simulink model "MyoGesture6CH_UI"  (R2018b)
settings: Solver=VariableStepAuto  StartTime=0.0  StopTime=inf  RelTol=1e-3
undefined symbols (not defined in the file or in its folder): serial
libraries: dspstat3 x8, instrumentlib x2, aerolibanimutils x1, dspnetwork x1
settings Model: Creator=Bruger  LastModifiedBy=anton

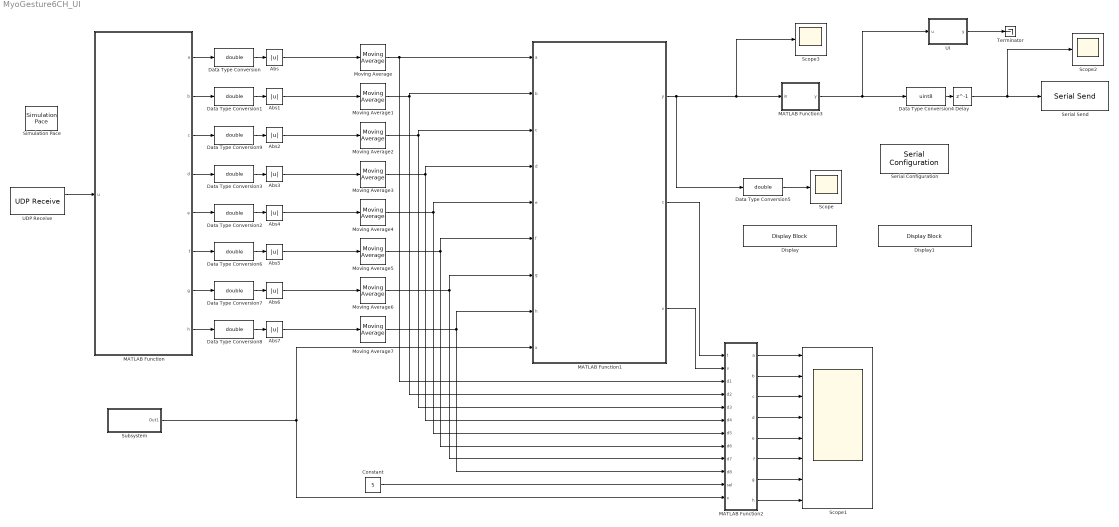
== system MyoGesture6CH_UI ==
  Abs{,1..7} (8 alike) : Abs
  Constant : Constant  Value=5
  Data Type Conversion{,1..3,5..9} (9 alike) : DataTypeConversion  OutDataTypeStr=double
  Data Type Conversion4 : DataTypeConversion  OutDataTypeStr=uint8
  Delay : Delay  DelayLength=1  InitialCondition=0
  Display : DisplayBlock  WebBlockId=99  LabelPosition=Hide
  Display1 : DisplayBlock  WebBlockId=154  LabelPosition=Hide
  MATLAB Function : MATLAB Function  TreatAsAtomicUnit=on
  MATLAB Function1 : MATLAB Function  TreatAsAtomicUnit=on
  MATLAB Function2 : MATLAB Function  TreatAsAtomicUnit=on
  MATLAB Function3 : MATLAB Function  TreatAsAtomicUnit=on
  Moving Average{,1..7} (8 alike) : dspstat3/Moving Average  Method=Sliding window  ForgettingFactorPort=off  SpecifyWindowLength=on  WindowLength=50  ForgettingFactor=0.9  SimulateUsing=Code generation
  Scope : Scope
  Scope1 : Scope  NumInputPorts=8
  Scope2 : Scope
  Scope3 : Scope
  Serial Configuration : instrumentlib/Serial Configuration  Priority=-200000  ComPortMenu=COM13  ComPort=COM13  ObjConstructor=serial('COM13');  BaudRate=12000000  DataBits=8  Parity=none  StopBits=1  FlowControl=none  Timeout=10  ByteOrder=LittleEndian
  Serial Send : instrumentlib/Serial Send  ComPortMenu=COM13  ComPort=COM13  ObjConstructor=serial('COM13');  Terminator=<none>  EnableBlockingMode=on
  Simulation Pace : aerolibanimutils/Simulation Pace  SimulationPace=1  SleepMode=Auto  OutputPaceError=off  SampleTime=1/30
  Subsystem : Subsystem
  Terminator : Terminator
  UDP Receive : dspnetwork/UDP Receive  localURL='0.0.0.0'  localPort=54000  remoteURL='0.0.0.0'  remotePort=-1  recvBufferSize=32  dims=255  signalDatatype=int8  isVarSize=off  showBlockingTime=off  blockingTime=0  sampletime=0.02  blockPlatform=[]
      settings: SourceProductName=DSP System Toolbox  SourceProductBaseCode=DS
  UI : MATLAB Function  Tag=rand  TreatAsAtomicUnit=on
  wires:
  UDP Receive/1 -> MATLAB Function/1(u)
  MATLAB Function/1(a) -> Data Type Conversion/1
  Data Type Conversion1/1 -> Abs1/1
  MATLAB Function/2(b) -> Data Type Conversion1/1
  Data Type Conversion2/1 -> Abs4/1
  Data Type Conversion3/1 -> Abs3/1
  Data Type Conversion6/1 -> Abs5/1
  Data Type Conversion7/1 -> Abs6/1
  Data Type Conversion8/1 -> Abs7/1
  Data Type Conversion9/1 -> Abs2/1
  MATLAB Function/8(h) -> Data Type Conversion8/1
  MATLAB Function/7(g) -> Data Type Conversion7/1
  MATLAB Function/6(f) -> Data Type Conversion6/1
  MATLAB Function/5(e) -> Data Type Conversion2/1
  MATLAB Function/4(d) -> Data Type Conversion3/1
  MATLAB Function/3(c) -> Data Type Conversion9/1
  Abs1/1 -> Moving Average1/1
  Abs7/1 -> Moving Average7/1
  Abs6/1 -> Moving Average6/1
  Abs5/1 -> Moving Average5/1
  Abs4/1 -> Moving Average4/1
  Abs3/1 -> Moving Average3/1
  Abs2/1 -> Moving Average2/1
  Moving Average1/1 -> MATLAB Function2/4(d2), MATLAB Function1/2(b)
  Moving Average2/1 -> MATLAB Function2/5(d3), MATLAB Function1/3(c)
  Moving Average3/1 -> MATLAB Function2/6(d4), MATLAB Function1/4(d)
  Moving Average4/1 -> MATLAB Function2/7(d5), MATLAB Function1/5(e)
  Moving Average5/1 -> MATLAB Function2/8(d6), MATLAB Function1/6(f)
  Moving Average6/1 -> MATLAB Function2/9(d7), MATLAB Function1/7(g)
  Moving Average7/1 -> MATLAB Function2/10(d8), MATLAB Function1/8(h)
  Data Type Conversion/1 -> Abs/1
  Abs/1 -> Moving Average/1
  Moving Average/1 -> MATLAB Function2/3(d1), MATLAB Function1/1(a)
  Subsystem/1(Out1) -> MATLAB Function1/9(x), MATLAB Function2/12(x)
  Constant/1 -> MATLAB Function2/11(sel)
  MATLAB Function2/8(h) -> Scope1/8
  MATLAB Function2/7(g) -> Scope1/7
  MATLAB Function2/1(a) -> Scope1/1
  MATLAB Function2/2(b) -> Scope1/2
  MATLAB Function2/3(c) -> Scope1/3
  MATLAB Function2/4(d) -> Scope1/4
  MATLAB Function2/5(e) -> Scope1/5
  MATLAB Function2/6(f) -> Scope1/6
  MATLAB Function1/2(t) -> MATLAB Function2/1(t)
  MATLAB Function1/3(v) -> MATLAB Function2/2(v)
  Data Type Conversion5/1 -> Scope/1
  Data Type Conversion4/1 -> Delay/1
  MATLAB Function1/1(y) -> Data Type Conversion5/1, Scope3/1, MATLAB Function3/1(in)
  Delay/1 -> Scope2/1, Serial Send/1
  MATLAB Function3/1(y) -> UI/1(u), Data Type Conversion4/1
  UI/1(y) -> Terminator/1

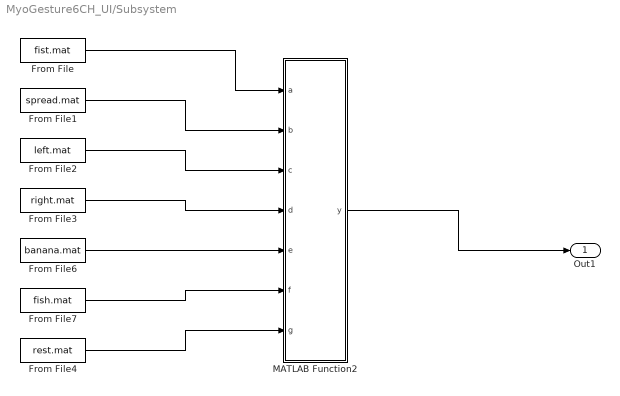
== system MyoGesture6CH_UI/Subsystem ==
  From File : FromFile  FileName=fist.mat  OutDataTypeStr=double  SampleTime=0  ExtrapolationBeforeFirstDataPoint=Hold first value  InterpolationWithinTimeRange=Zero order hold  ExtrapolationAfterLastDataPoint=Hold last value
  From File1 : FromFile  FileName=spread.mat  OutDataTypeStr=double  SampleTime=0  ExtrapolationBeforeFirstDataPoint=Hold first value  InterpolationWithinTimeRange=Zero order hold  ExtrapolationAfterLastDataPoint=Hold last value
  From File2 : FromFile  FileName=left.mat  OutDataTypeStr=double  SampleTime=0  ExtrapolationBeforeFirstDataPoint=Hold first value  InterpolationWithinTimeRange=Zero order hold  ExtrapolationAfterLastDataPoint=Hold last value
  From File3 : FromFile  FileName=right.mat  OutDataTypeStr=double  SampleTime=0  ExtrapolationBeforeFirstDataPoint=Hold first value  InterpolationWithinTimeRange=Zero order hold  ExtrapolationAfterLastDataPoint=Hold last value
  From File4 : FromFile  FileName=rest.mat  OutDataTypeStr=double  SampleTime=0  ExtrapolationBeforeFirstDataPoint=Hold first value  InterpolationWithinTimeRange=Zero order hold  ExtrapolationAfterLastDataPoint=Hold last value
  From File6 : FromFile  FileName=banana.mat  OutDataTypeStr=double  SampleTime=0  ExtrapolationBeforeFirstDataPoint=Hold first value  InterpolationWithinTimeRange=Zero order hold  ExtrapolationAfterLastDataPoint=Hold last value
  From File7 : FromFile  FileName=fish.mat  OutDataTypeStr=double  SampleTime=0  ExtrapolationBeforeFirstDataPoint=Hold first value  InterpolationWithinTimeRange=Zero order hold  ExtrapolationAfterLastDataPoint=Hold last value
  MATLAB Function2 : MATLAB Function  TreatAsAtomicUnit=on
  Out1 : Outport
  wires:
  MATLAB Function2/1(y) -> Out1/1
  From File/1 -> MATLAB Function2/1(a)
  From File6/1 -> MATLAB Function2/5(e)
  From File1/1 -> MATLAB Function2/2(b)
  From File7/1 -> MATLAB Function2/6(f)
  From File3/1 -> MATLAB Function2/4(d)
  From File2/1 -> MATLAB Function2/3(c)
  From File4/1 -> MATLAB Function2/7(g)

== matlab function MyoGesture6CH_UI/MATLAB Function1 ==
  data: a input; y output; b input; c input; d input; e input; f input; g input; h input; x input; t output; v output
function [y,t,v] = fcn(a,b,c,d,e,f,g,h,x)

%Percentage
t = 1.5; %top
v = 0.6; %bot

%constant
n = 1;  %top
m = 0;  %bot

    if a<x(1,7)*t+n & a>x(2,7)*v-m & b<x(3,7)*t+n & b>x(4,7)*v-m & c<x(5,7)*t+n & c>x(6,7)*v-m & d<x(7,7)*t+n & d>x(8,7)*v-m & e<x(9,7)*t+n & e>x(10,7)*v-m & f<x(11,7)*t+n & f>x(12,7)*v-m & g<x(13,7)*t+n & g>x(14,7)*v-m & h<x(15,7)*t+n & h>x(16,7)*v-m 
        y=0;
    elseif a<x(1,1)*t+n & a>x(2,1)*v-m & b<x(3,1)*t+n & b>x(4,1)*v-m & c<x(5,1)*t+n & c>x(6,1)*v-m & d<x(7,1)*t+n & d>x(8,1)*v-m & e<x(9,1)*t+n & e>x(10,1)*v-m & f<x(11,1)*t+n & f>x(12,1)*v-m & g<x(13,1)*t+n & g>x(14,1)*v-m & h<x(15,1)*t+n & h>x(16,1)*v-m 
        y=1;
    elseif a<x(1,2)*t+n & a>x(2,2)*v-m & b<x(3,2)*t+n & b>x(4,2)*v-m & c<x(5,2)*t+n & c>x(6,2)*v-m & d<x(7,2)*t+n & d>x(8,2)*v-m & e<x(9,2)*t+n & e>x(10,2)*v-m & f<x(11,2)*t+n & f>x(12,2)*v-m & g<x(13,2)*t+n & g>x(14,2)*v-m & h<x(15,2)*t+n & h>x(16,2)*v-m 
        y=2;
    elseif a<x(1,3)*t+n & a>x(2,3)*v-m & b<x(3,3)*t+n & b>x(4,3)*v-m & c<x(5,3)*t+n & c>x(6,3)*v-m & d<x(7,3)*t+n & d>x(8,3)*v-m & e<x(9,3)*t+n & e>x(10,3)*v-m & f<x(11,3)*t+n & f>x(12,3)*v-m & g<x(13,3)*t+n & g>x(14,3)*v-m & h<x(15,3)*t+n & h>x(16,3)*v-m 
        y=3;
    elseif a<x(1,4)*t+n & a>x(2,4)*v-m & b<x(3,4)*t+n & b>x(4,4)*v-m & c<x(5,4)*t+n & c>x(6,4)*v-m & d<x(7,4)*t+n & d>x(8,4)*v-m & e<x(9,4)*t+n & e>x(10,4)*v-m & f<x(11,4)*t+n & f>x(12,4)*v-m & g<x(13,4)*t+n & g>x(14,4)*v-m & h<x(15,4)*t+n & h>x(16,4)*v-m 
        y=4;
    elseif a<x(1,5)*t+n & a>x(2,5)*v-m & b<x(3,5)*t+n & b>x(4,5)*v-m & c<x(5,5)*t+n & c>x(6,5)*v-m & d<x(7,5)*t+n & d>x(8,5)*v-m & e<x(9,5)*t+n & e>x(10,5)*v-m & f<x(11,5)*t+n & f>x(12,5)*v-m & g<x(13,5)*t+n & g>x(14,5)*v-m & h<x(15,5)*t+n & h>x(16,5)*v-m 
        y=5;
%     elseif a<x(1,6)*t+n & a>x(2,6)*v-m & b<x(3,6)*t+n & b>x(4,6)*v-m & c<x(5,6)*t+n & c>x(6,6)*v-m & d<x(7,6)*t+n & d>x(8,6)*v-m & e<x(9,6)*t+n & e>x(10,6)*v-m & f<x(11,6)*t+n & f>x(12,6)*v-m & g<x(13,6)*t+n & g>x(14,6)*v-m & h<x(15,6)*t+n & h>x(16,6)*v-m 
%         y=6;
               
    else
y=0
    
    end

% %Threshold with Addition
% t = 9;
% v = 3;
% 
%     if a<x(1,1)+t & a>x(2,1)-v & b<x(3,1)+t & b>x(4,1)-v & c<x(5,1)+t & c>x(6,1)-v & d<x(7,1)+t & d>x(8,1)-v & e<x(9,1)+t & e>x(10,1)-v & f<x(11,1)+t & f>x(12,1)-v & g<x(13,1)+t & g>x(14,1)-v & h<x(15,1)+t & h>x(16,1)-v 
%         y=1;
%     elseif a<x(1,2)+t & a>x(2,2)-v & b<x(3,2)+t & b>x(4,2)-v & c<x(5,2)+t & c>x(6,2)-v & d<x(7,2)+t & d>x(8,2)-v & e<x(9,2)+t & e>x(10,2)-v & f<x(11,2)+t & f>x(12,2)-v & g<x(13,2)+t & g>x(14,2)-v & h<x(15,2)+t & h>x(16,2)-v 
%         y=2;
%     elseif a<x(1,3)+t & a>x(2,3)-v & b<x(3,3)+t & b>x(4,3)-v & c<x(5,3)+t & c>x(6,3)-v & d<x(7,3)+t & d>x(8,3)-v & e<x(9,3)+t & e>x(10,3)-v & f<x(11,3)+t & f>x(12,3)-v & g<x(13,3)+t & g>x(14,3)-v & h<x(15,3)+t & h>x(16,3)-v 
%         y=3;
%     elseif a<x(1,4)+t & a>x(2,4)-v & b<x(3,4)+t & b>x(4,4)-v & c<x(5,4)+t & c>x(6,4)-v & d<x(7,4)+t & d>x(8,4)-v & e<x(9,4)+t & e>x(10,4)-v & f<x(11,4)+t & f>x(12,4)-v & g<x(13,4)+t & g>x(14,4)-v & h<x(15,4)+t & h>x(16,4)-v 
%         y=4;
%     elseif a<x(1,5)+t & a>x(2,5)-v & b<x(3,5)+t & b>x(4,5)-v & c<x(5,5)+t & c>x(6,5)-v & d<x(7,5)+t & d>x(8,5)-v & e<x(9,5)+t & e>x(10,5)-v & f<x(11,5)+t & f>x(12,5)-v & g<x(13,5)+t & g>x(14,5)-v & h<x(15,5)+t & h>x(16,5)-v 
%         y=5;
%     elseif a<x(1,6)+t & a>x(2,6)-v & b<x(3,6)+t & b>x(4,6)-v & c<x(5,6)+t & c>x(6,6)-v & d<x(7,6)+t & d>x(8,6)-v & e<x(9,6)+t & e>x(10,6)-v & f<x(11,6)+t & f>x(12,6)-v & g<x(13,6)+t & g>x(14,6)-v & h<x(15,6)+t & h>x(16,6)-v 
%         y=6;
%     elseif a<x(1,7)+t & a>x(2,7)-v & b<x(3,7)+t & b>x(4,7)-v & c<x(5,7)+t & c>x(6,7)-v & d<x(7,7)+t & d>x(8,7)-v & e<x(9,7)+t & e>x(10,7)-v & f<x(11,7)+t & f>x(12,7)-v & g<x(13,7)+t & g>x(14,7)-v & h<x(15,7)+t & h>x(16,7)-v 
%         y=7;
%     elseif a<x(1,8)+t & a>x(2,8)-v & b<x(3,8)+t & b>x(4,8)-v & c<x(5,8)+t & c>x(6,8)-v & d<x(7,8)+t & d>x(8,8)-v & e<x(9,8)+t & e>x(10,8)-v & f<x(11,8)+t & f>x(12,8)-v & g<x(13,8)+t & g>x(14,8)-v & h<x(15,8)+t & h>x(16,8)-v 
%         y=8;
%             
%     else
% y=0
%     
%     end

== matlab function MyoGesture6CH_UI/MATLAB Function ==
  data: u input; a output; b output; c output; d output; e output; f output; g output; h output
%a is the output of this block, and fcn(u) is the input required
function [a,b,c,d,e,f,g,h]  = fcn(u)
        
%Below the output a is specified as the 3 row of the 8x1 input vector u
a = u(1,:);
b = u(2,:);
c = u(3,:);
d = u(4,:);
e = u(5,:);
f = u(6,:);
g = u(7,:);
h = u(8,:);

== matlab function MyoGesture6CH_UI/MATLAB Function2 ==
  data: t input; v input; d1 input; d2 input; d3 input; d4 input; d5 input; d6 input; d7 input; d8 input; sel input; x input; a output; b output; c output; d output; e output; f output; g output; h output
function [a,b,c,d,e,f,g,h] = fcn(t, v, d1, d2, d3, d4, d5, d6, d7, d8, sel, x)
    
    a=[x(1,sel)*t*t,x(2,sel)*v,d1]
    b=[x(3,sel)*t,x(4,sel)*v,d2]
    c=[x(5,sel)*t,x(6,sel)*v,d3]
    d=[x(7,sel)*t,x(8,sel)*v,d4]
    e=[x(9,sel)*t,x(10,sel)*v,d5]
    f=[x(11,sel)*t,x(12,sel)*v,d6]
    g=[x(13,sel)*t,x(14,sel)*v,d7]
    h=[x(15,sel)*t,x(16,sel)*v,d8]

== matlab function MyoGesture6CH_UI/Subsystem/MATLAB Function2 ==
  data: a input; b input; c input; d input; e input; f input; g input; y output
function y = fcn(a, b, c, d, e, f, g)

y=[a b c d e f g];

== matlab function MyoGesture6CH_UI/MATLAB Function3 ==
  data: in input; y output
function y = fcn(in)

persistent A;
if isempty(A)
    A=zeros(1,150);
end

if in==0
    A=zeros(1,150);
end

    A=circshift(A,1);
    A(1)=in;   
    M = mode(A)

y = M;

== matlab function MyoGesture6CH_UI/UI ==
  data: u input; y output
function y = fcn(u)
coder.extrinsic('uicontrol');
coder.extrinsic('uipanel');

persistent h1 h5 h6 prev jointUp jointDown selected; 
% persistent h1 h5 prev;

if isempty(prev)
    prev=0;
end

if isempty(jointUp)
    jointUp=0;
    jointDown=0;
    selected=1;
end

if isempty(h1) 
     close all;
     h1 = figure(...
    'PaperUnits','inches',...
    'Units','characters',...
    'Position',[100 10 120 35],...
    'Name','UI',...
    'PaperSize',[8.5 11]); 

    h2 = uipanel(...
    'Parent',h1,...
    'FontSize',10,...
    'Units','characters',...
    'Title','Instructions',...
    'Position',[55.8 19.0769230769231 59 11.6153846153846]);

    h3 = uicontrol(...
    'Parent',h2,...
    'Units','characters',...
    'HorizontalAlignment','left',...
    'String',{  'SPREAD: open/close gripper	'; 'WAVE LEFT: move joint counter-clockwise	'; 'WAVE RIGHT: move joint clockwise 	'; 'FIST PULL-BACK: joint select up	'; 'FIST: joint select down 	'; 'RELAXED: stop command	' },...
    'Style','text',...
    'Position',[3.4 1.61538461538462 50 8],...
    'FontSize',10); 

%     'FontSize',10,...
%     'FontWeight','bold');

%     h4 = uicontrol(...
%     'Parent',h2,...
%     'Units','characters',...
%     'HorizontalAlignment','left',...
%     'String',{  'open/close gripper '; 'move joint counter-clockwise'; 'move joint clockwise '; 'joint select up'; 'joint select down'; 'stop command' },...
%     'Style','text',...
%     'Position',[23.4 1.61538461538462 28.8 8],...
%     'FontSize',12);

    h5 = uipanel(...
    'Parent',h1,...
    'FontSize',10,...
    'Units','characters',...
    'Title','Current gesture',...
    'Position',[9.8 25 42.2 5.69230769230769]);

    h6 = uipanel(...
    'Parent',h1,...
    'FontSize',10,...
    'Units','characters',...
    'Title','Selected joint',...
    'Position',[9.8 18.5 42.2 5.69230769230769]);

    h7 = uicontrol(...
    'Parent',h5,...
    'Units','characters',...
    'String',{ 'Relaxed' },...
    'Style','text',...
    'Position',[3 1 36.8 2.38461538461538],...
    'FontSize',10);

    h8 = uicontrol(...
    'Parent',h6,...
    'Units','characters',...
    'String',{ '1' },...
    'Style','text',...
    'Position',[3 1 36.8 2.38461538461538],...
    'FontSize',10);
% %     
end
% 
% % % % % % % % % % % % % % % % % % % % % % % % % % % % % % % % % % % % % % % % % % % % % % % % % % 
% % % % % % % % % % % % % % % % % % % % % % % % % % % % % % % % % % % % % % % % % % % % % % % % % % 
% % % % % % % % % % % % % % % % % % % % % % % % % % % % % % % % % % % % % % % % % % % % % % % % % % 
% 
if u==4
    jointUp=jointUp+1;   
    if jointUp>150
        jointUp=0;
    end
else
    jointUp=0;
end

if u==5
    jointDown=jointDown+1;  
    if jointDown>150
        jointDown=0;
    end   
else
    jointDown=0;
end
% % 
if jointUp==5 || jointUp==150
    if selected~=3
        h8 = uicontrol(...
        'Parent',h6,...
        'Units','characters',...
        'String',{ selected+1 },...
        'Style','text',...
        'Position',[3 1 36.8 2.38461538461538],...
        'FontSize',10);
    
        selected=selected+1;
        
    else
        h8 = uicontrol(...
        'Parent',h6,...
        'Units','characters',...
        'String',{'3' },...
        'Style','text',...
        'Position',[3 1 36.8 2.38461538461538],...
        'FontSize',10);
    end
end
        
if jointDown==5 || jointDown==150
    if selected~=1
        h8 = uicontrol(...
        'Parent',h6,...
        'Units','characters',...
        'String',{ selected-1 },...
        'Style','text',...
        'Position',[3 1 36.8 2.38461538461538],...
        'FontSize',10);
    
        selected=selected-1; 
    else
        h8 = uicontrol(...
        'Parent',h6,...
        'Units','characters',...
        'String',{ '1' },...
        'Style','text',...
        'Position',[3 1 36.8 2.38461538461538],...
        'FontSize',10);
    end
end
% 

if u~=prev
    switch u
        case 1
            output='Spread';
            prev=1;
        case 2
            output='Wave Left';
            prev=2;
        case 3
            output='Wave Right';
            prev=3;
        case 4
            output='Fist Pull-back';
            prev=4;
        case 5
            output='Fist';
            prev=5;
        case 0
            output='Relaxed';
            prev=0;
        otherwise
            output='Error';
    end

      h7 = uicontrol(...
        'Parent',h5,...
        'Units','characters',...
        'String',{ output },...
        'Style','text',...
        'Position',[3 1 36.8 2.38461538461538],...
        'FontSize',10);
end

y = u;
